simulink model "ejemplo02"  (R2021b)
settings: Solver=VariableStepAuto  StartTime=1  StopTime=10.0  RelTol=1e-3
settings Model: Creator=juandiegocastropadilla  LastModifiedBy=juandiegocastropadilla

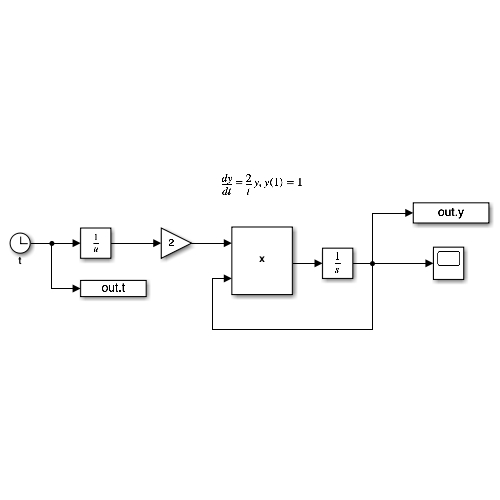
[thumbnail: Simulink's stored preview of the top-level diagram]
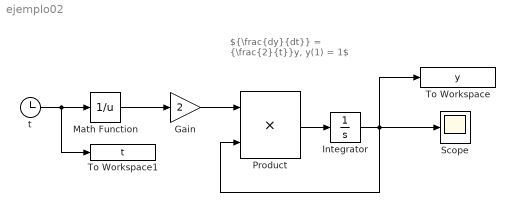
== system ejemplo02 ==
  note: ${\frac{dy}{dt}} = {\frac{2}{t}}y, y(1) = 1$
  Gain : Gain  Gain=2
  Integrator : Integrator  InitialCondition=1
  Math Function : Math  Operator=reciprocal  SaturateOnIntegerOverflow=on
  Product : Product
  Scope : Scope
  To Workspace : ToWorkspace  VariableName=y  SampleTime=-1
  To Workspace1 : ToWorkspace  VariableName=t  SampleTime=-1
  t : Clock
  wires:
  Math Function/1 -> Gain/1
  Gain/1 -> Product/1
  Product/1 -> Integrator/1
  Integrator/1 -> To Workspace/1, Scope/1, Product/2
  t/1 -> To Workspace1/1, Math Function/1
